simulink model "Rete"  (Simulink 9.0)
settings: Solver=VariableStepAuto  StartTime=0.0  StopTime=7200  RelTol=1e-3
values from neighbouring files (symbols this model uses):
  r_pompa = 100    [Circuit_configurator.m]
  vasca_1_r = 100    [Circuit_configurator.m]
  vasca_2_r = 100    [Circuit_configurator.m]
  vasca_3_r = 100    [Circuit_configurator.m]
  vasca_r_in = single(100)    [Circuit_configurator.m]
  vasca_sw = uint8(1)    [Circuit_configurator.m]
libraries: fl_lib x27, nesl_utility x24, elec_lib x8, realtime_pacer_lib x1
settings Model: SuppressorTable=22 serialization::archive 11 0 6 0 0 0 11 0  Creator=aleskandro  LastModifiedBy=aleskandro
settings DataIOCC: SaveFormat=Dataset
settings OptimizationCC: LifeSpan=auto
settings DebuggingCC: UnderspecifiedInitializationDetection=Simplified  MergeDetectMultiDrivingBlocksExec=error  SFUnexpectedBacktrackingDiag=error  SFNoUnconditionalDefaultTransitionDiag=error  SFExecutionAtInitializationDiag=warning
settings HardwareCC: ProdBitPerPointer=64  ProdBitPerSizeT=64  ProdBitPerPtrDiffT=64  ProdLargestAtomicFloat=Float  ProdIntDivRoundTo=Zero  ProdEndianess=LittleEndian  ProdWordSize=64  ProdHWDeviceType=Intel->x86-64 (Windows64)
settings ModelReferenceCC: PropagateSignalLabelsOutOfModel=on
settings GRTTargetCC: TargetLangStandard=C99 (ISO)
settings ConfigComp: CovMetricSettings=dwe  CovHtmlReporting=off  CovSaveCumulativeToWorkspaceVar=off  CovSaveSingleToWorkspaceVar=off  CovExternalEMLEnable=on
settings SimscapeCC: SimscapeNormalizeSystem=off

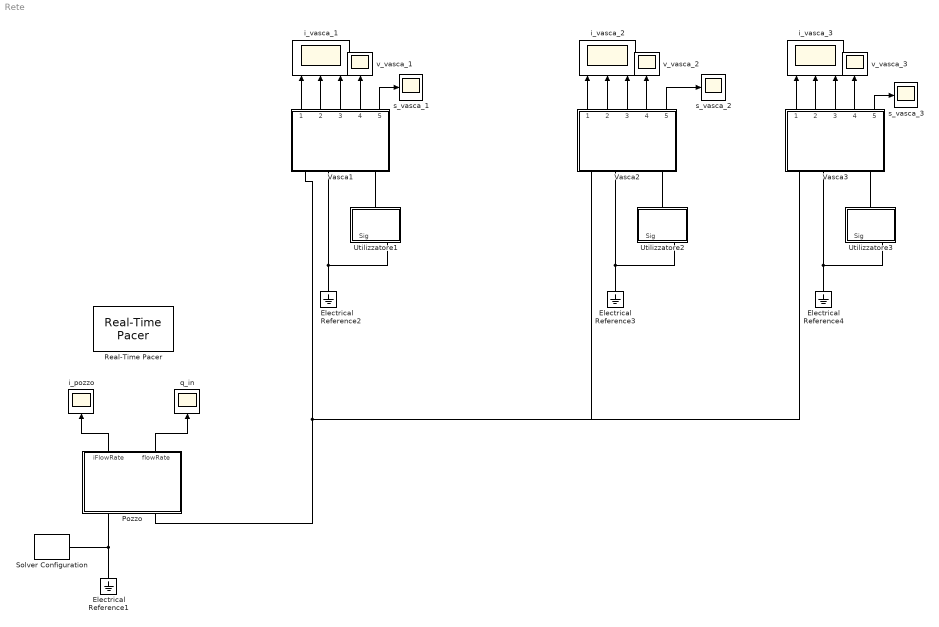
== system Rete ==
  Electrical Reference{1..4} (4 alike) : fl_lib/Electrical/Electrical Elements/Electrical Reference
  Pozzo : Subsystem
  Real-Time Pacer : realtime_pacer_lib/Real-Time Pacer  simTimePerRealTime=1
  Solver Configuration : nesl_utility/Solver Configuration  PhysicalDomain=network_engine_domain  SubClassName=solver  LeftPortType=input  RightPortType=generic  Accelerate=off  Tones=[]  Harmonics=[]  SimulateNoise=off  Profile=off  UseLocalSampling=off  EnableSwitchedLinearOptims=on  FrequencyDomain=off  UseCCode=off  RelTol=0.001  AbsTol=1e-06  MinStep=1e-09  ToWorkspace=off  RevertToSquareIcSolve=off  NumHomotopyIterations=100  PhasorMode=off  PhasorModeNumHarmonics=1  DoDC=off  ResidualTolerance=1e-09  UseLocalSolver=on  LocalSolverChoice=NE_BACKWARD_EULER_ADVANCER  LocalSolverSampleTime=0.1  DoFixedCost=on  MaxNonlinIter=3  MaxModeIter=2  LinearAlgebra=Sparse  DelaysMemoryBudget=1024  AutomaticFiltering=on  FilteringTimeConstant=0.001
  Utilizzatore1 : Subsystem
  Utilizzatore2 : Subsystem
  Utilizzatore3 : Subsystem
  Vasca1 : Subsystem
  Vasca2 : Subsystem
  Vasca3 : Subsystem
  i_pozzo : Scope
  i_vasca_1 : Scope  NumInputPorts=3
  i_vasca_2 : Scope  NumInputPorts=3
  i_vasca_3 : Scope  NumInputPorts=3
  q_in : Scope
  s_vasca_1 : Scope
  s_vasca_2 : Scope
  s_vasca_3 : Scope
  v_vasca_1 : Scope
  v_vasca_2 : Scope
  v_vasca_3 : Scope
  wires:
  Vasca1/4(vPression) -> v_vasca_1/1
  Pozzo/2(flowRate) -> q_in/1
  Pozzo/1(iFlowRate) -> i_pozzo/1
  Vasca1/2(flowRateOut) -> i_vasca_1/2
  Vasca1/1(flowRateIn) -> i_vasca_1/1
  Vasca1/3(vFlowRate) -> i_vasca_1/3
  Vasca2/3(vFlowRate) -> i_vasca_2/3
  Vasca2/4(vPression) -> v_vasca_2/1
  Vasca2/2(flowRateOut) -> i_vasca_2/2
  Vasca2/1(flowRateIn) -> i_vasca_2/1
  Vasca3/3(vFlowRate) -> i_vasca_3/3
  Vasca3/4(vPression) -> v_vasca_3/1
  Vasca3/2(flowRateOut) -> i_vasca_3/2
  Vasca3/1(flowRateIn) -> i_vasca_3/1
  Vasca2/5(switch) -> s_vasca_2/1
  Vasca3/5(switch) -> s_vasca_3/1
  Vasca1/5(switch) -> s_vasca_1/1
  connections:
  Electrical Reference1/LConn1 -- Solver Configuration/RConn1 -- Pozzo/LConn1
  Electrical Reference2/LConn1 -- Utilizzatore1/RConn1 -- Vasca1/LConn2
  Vasca1/LConn4 -- Utilizzatore1/LConn1
  Electrical Reference3/LConn1 -- Vasca2/LConn2 -- Utilizzatore2/RConn1
  Vasca2/LConn4 -- Utilizzatore2/LConn1
  Electrical Reference4/LConn1 -- Vasca3/LConn2 -- Utilizzatore3/RConn1
  Vasca3/LConn4 -- Utilizzatore3/LConn1
  Vasca3/LConn1 -- Vasca2/LConn1 -- Pozzo/LConn2 -- Vasca1/LConn1

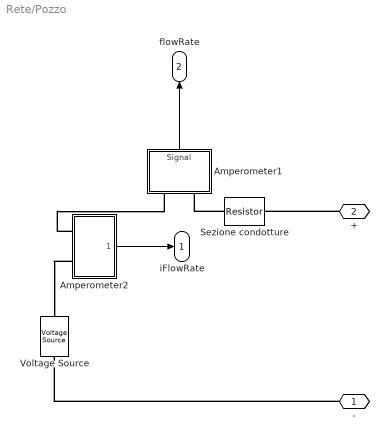
== system Rete/Pozzo ==
  Amperometer1 : Subsystem
  Amperometer2 : Subsystem
  Sezione condotture : elec_lib/Passive Devices/Resistor  R=r_pompa Ohm  R_tol=5  enable_R_tol=0  tol_distribution=1  nSigma=4  enable_operating_limits=0  operating_limit_action=2  max_working_voltage=100 V  power_rating=1 W  enable_faults=0  fault_action=1  R_faulted=Inf Ohm  enable_temporal_fault=0  t_fault=1 s  enable_behavioral_fault=0  max_permissible_current=1 A  t_fail_on_current=1 s  noise_mode=0  sample_time=0.001 s  repeatability=1  auto_seed=3797408467  user_seed=0  Tdevice=25 degC  alpha=3.93e-3 1/K  Tmeas=25 degC  thermal_mass=100 J/K  power_derating_T1=70 degC  power_derating_T2=155 degC  operating_temperature_range_vec=[-50, 150] degC  temperature_specify=off  temperature_priority=High  temperature=298.15 K  temperature_nominal_specify=off  temperature_nominal_unit=K  temperature_nominal_value=1
  Voltage Source : elec_lib/Sources/Voltage Source  dc_voltage=v_pompa V  ac_voltage=0 V  ac_shift=0 deg  ac_frequency=0 Hz  noise_mode=0  PSD=0 V^2/Hz  repeatability=1  auto_seed=2589191353  user_seed=0  sample_time=0.001 s  i_specify=off  i_priority=None  i=0 A  i_nominal_specify=off  i_nominal_unit=A  i_nominal_value=1  v_specify=off  v_priority=None  v=0 V  v_nominal_specify=off  v_nominal_unit=V  v_nominal_value=1
      settings: SourceProductName=Simscape Electronics  SourceProductBaseCode=SN
  - : PMIOPort  Port=1  Side=Left
  + : PMIOPort  Port=2  Side=Left
  iFlowRate : Outport
  flowRate : Outport  Port=2
  wires:
  Amperometer2/1(Signal) -> iFlowRate/1
  Amperometer1/1(Signal) -> flowRate/1
  connections:
  +/RConn1 -- Sezione condotture/RConn1
  -/RConn1 -- Voltage Source/RConn1
  Amperometer2/LConn2 -- Voltage Source/LConn1
  Amperometer2/LConn1 -- Amperometer1/LConn1
  Sezione condotture/LConn1 -- Amperometer1/LConn2

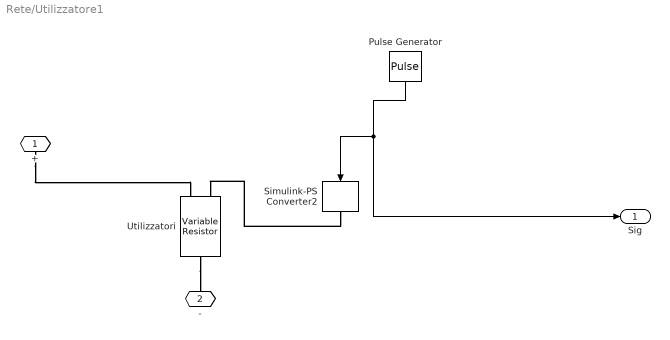
== system Rete/Utilizzatore1 ==
  Pulse Generator : DiscretePulseGenerator  Amplitude=999999999  Period=3000  PulseWidth=1500  PhaseDelay=4200
  Simulink-PS Converter2 : nesl_utility/Simulink-PS Converter  PhysicalDomain=network_engine_domain  SubClassName=ps_input  LeftPortType=input  RightPortType=output  PseudoPeriodic=off  Frequencies=[]  NoiseDistribution=none  NoiseParameters=[]  Unit=1  AffineConversion=off  FilteringAndDerivatives=zero  SimscapeFilterOrder=1  InputFilterTimeConstant=0.001  UdotUserProvided=1
  Utilizzatori : fl_lib/Electrical/Electrical Elements/Variable Resistor  Rmin=0 Ohm  i_specify=off  i_priority=High  i=0 A  i_nominal_specify=off  i_nominal_unit=A  i_nominal_value=1  v_specify=off  v_priority=High  v=0 V  v_nominal_specify=off  v_nominal_unit=V  v_nominal_value=1
  + : PMIOPort  Port=1  Side=Left
  - : PMIOPort  Port=2  Side=Right
  Sig : Outport
  wires:
  Pulse Generator/1 -> Sig/1, Simulink-PS Converter2/1
  connections:
  +/RConn1 -- Utilizzatori/LConn2
  Utilizzatori/RConn1 -- -/RConn1
  Simulink-PS Converter2/RConn1 -- Utilizzatori/LConn1

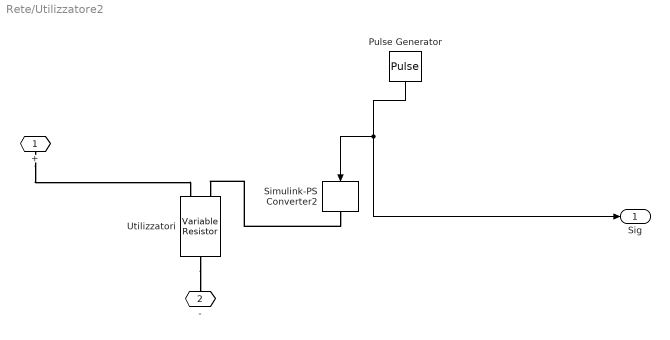
== system Rete/Utilizzatore2 ==
  Pulse Generator : DiscretePulseGenerator  Amplitude=999999999  Period=3000  PulseWidth=1500  PhaseDelay=4200
  Simulink-PS Converter2 : nesl_utility/Simulink-PS Converter  PhysicalDomain=network_engine_domain  SubClassName=ps_input  LeftPortType=input  RightPortType=output  PseudoPeriodic=off  Frequencies=[]  NoiseDistribution=none  NoiseParameters=[]  Unit=1  AffineConversion=off  FilteringAndDerivatives=zero  SimscapeFilterOrder=1  InputFilterTimeConstant=0.001  UdotUserProvided=1
  Utilizzatori : fl_lib/Electrical/Electrical Elements/Variable Resistor  Rmin=0 Ohm  i_specify=off  i_priority=High  i=0 A  i_nominal_specify=off  i_nominal_unit=A  i_nominal_value=1  v_specify=off  v_priority=High  v=0 V  v_nominal_specify=off  v_nominal_unit=V  v_nominal_value=1
  + : PMIOPort  Port=1  Side=Left
  - : PMIOPort  Port=2  Side=Right
  Sig : Outport
  wires:
  Pulse Generator/1 -> Sig/1, Simulink-PS Converter2/1
  connections:
  +/RConn1 -- Utilizzatori/LConn2
  Utilizzatori/RConn1 -- -/RConn1
  Simulink-PS Converter2/RConn1 -- Utilizzatori/LConn1

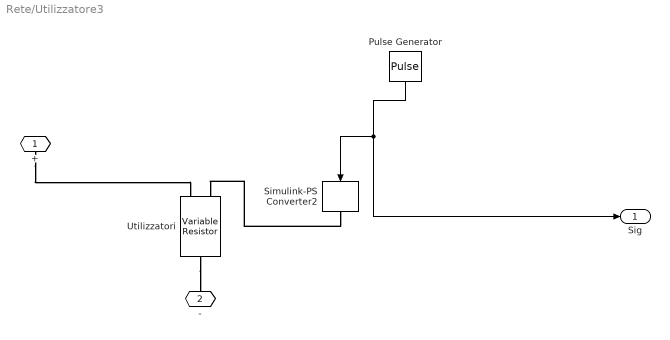
== system Rete/Utilizzatore3 ==
  Pulse Generator : DiscretePulseGenerator  Amplitude=999999999  Period=3000  PulseWidth=1500  PhaseDelay=4200
  Simulink-PS Converter2 : nesl_utility/Simulink-PS Converter  PhysicalDomain=network_engine_domain  SubClassName=ps_input  LeftPortType=input  RightPortType=output  PseudoPeriodic=off  Frequencies=[]  NoiseDistribution=none  NoiseParameters=[]  Unit=1  AffineConversion=off  FilteringAndDerivatives=zero  SimscapeFilterOrder=1  InputFilterTimeConstant=0.001  UdotUserProvided=1
  Utilizzatori : fl_lib/Electrical/Electrical Elements/Variable Resistor  Rmin=0 Ohm  i_specify=off  i_priority=High  i=0 A  i_nominal_specify=off  i_nominal_unit=A  i_nominal_value=1  v_specify=off  v_priority=High  v=0 V  v_nominal_specify=off  v_nominal_unit=V  v_nominal_value=1
  + : PMIOPort  Port=1  Side=Left
  - : PMIOPort  Port=2  Side=Right
  Sig : Outport
  wires:
  Pulse Generator/1 -> Sig/1, Simulink-PS Converter2/1
  connections:
  +/RConn1 -- Utilizzatori/LConn2
  Utilizzatori/RConn1 -- -/RConn1
  Simulink-PS Converter2/RConn1 -- Utilizzatori/LConn1

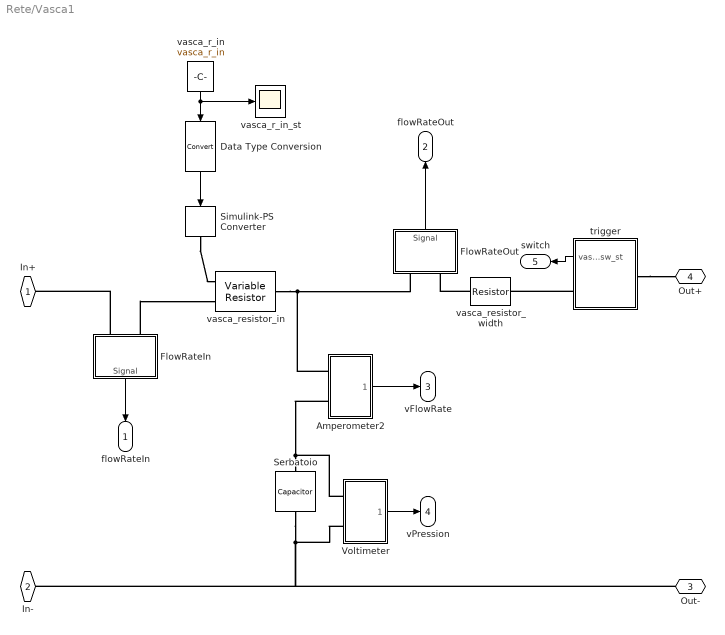
== system Rete/Vasca1 ==
  Amperometer2 : Subsystem
  Data Type Conversion : DataTypeConversion
  FlowRateIn : Subsystem
  FlowRateOut : Subsystem
  Serbatoio : elec_lib/Passive Devices/Capacitor  enable_table=0  c=vasca_1_c F  Cvec=[ 1e-5 1e-6 ] F  Vvec=[ 0 10 ] V  CV_table_symmetry=1  C_tol=5  enable_C_tol=0  tol_distribution=1  nSigma=4  r=1e-6 Ohm  g=0 1/Ohm  enable_operating_limits=0  operating_limit_action=2  max_working_voltage_range=[ -25 25 ] V  power_rating=1 W  enable_faults=0  fault_action=1  Cscale_faulted=100  R_faulted=0.001 Ohm  G_faulted=0 1/Ohm  tau_fault=0.001 s  enable_temporal_fault=0  t_fault=1 s  enable_behavioral_fault=0  max_permissible_voltage_range=[ -100 100 ] V  t_fail_on_voltage=1 s  i_specify=off  i_priority=None  i=0 A  i_nominal_specify=off  i_nominal_unit=A  i_nominal_value=1  v_specify=off  v_priority=None  v=0 V  v_nominal_specify=off  v_nominal_unit=V  v_nominal_value=1  vc_specify=on  vc_priority=High  vc=500 V  vc_nominal_specify=off  vc_nominal_unit=V  vc_nominal_value=1
  Simulink-PS Converter : nesl_utility/Simulink-PS Converter  PhysicalDomain=network_engine_domain  SubClassName=ps_input  LeftPortType=input  RightPortType=output  PseudoPeriodic=off  Frequencies=[]  NoiseDistribution=none  NoiseParameters=[]  Unit=1  AffineConversion=off  FilteringAndDerivatives=zero  SimscapeFilterOrder=1  InputFilterTimeConstant=0.001  UdotUserProvided=1
  Voltimeter : Subsystem
  trigger : Subsystem
  vasca_r_in : Constant  Value=vasca_r_in
  vasca_r_in_st : Scope
  vasca_resistor_in : fl_lib/Electrical/Electrical Elements/Variable Resistor  Rmin=0 Ohm  i_specify=off  i_priority=None  i=0 A  i_nominal_specify=off  i_nominal_unit=A  i_nominal_value=1  v_specify=off  v_priority=None  v=0 V  v_nominal_specify=off  v_nominal_unit=V  v_nominal_value=1
  vasca_resistor_width : elec_lib/Passive Devices/Resistor  R=vasca_1_r Ohm  R_tol=5  enable_R_tol=0  tol_distribution=1  nSigma=4  enable_operating_limits=0  operating_limit_action=2  max_working_voltage=100 V  power_rating=1 W  enable_faults=0  fault_action=1  R_faulted=Inf Ohm  enable_temporal_fault=0  t_fault=1 s  enable_behavioral_fault=0  max_permissible_current=1 A  t_fail_on_current=1 s  noise_mode=0  sample_time=0.001 s  repeatability=1  auto_seed=2536105935  user_seed=0  Tdevice=25 degC  alpha=3.93e-3 1/K  Tmeas=25 degC  thermal_mass=100 J/K  power_derating_T1=70 degC  power_derating_T2=155 degC  operating_temperature_range_vec=[-50, 150] degC  temperature_specify=off  temperature_priority=High  temperature=298.15 K  temperature_nominal_specify=off  temperature_nominal_unit=K  temperature_nominal_value=1
  In+ : PMIOPort  Port=1  Side=Left
  In- : PMIOPort  Port=2  Side=Left
  Out- : PMIOPort  Port=3  Side=Left
  Out+ : PMIOPort  Port=4  Side=Left
  flowRateIn : Outport
  flowRateOut : Outport  Port=2
  vFlowRate : Outport  Port=3
  vPression : Outport  Port=4
  switch : Outport  Port=5
  wires:
  Amperometer2/1(Signal) -> vFlowRate/1
  Voltimeter/1(Signal) -> vPression/1
  FlowRateOut/1(Signal) -> flowRateOut/1
  trigger/1(vasca_sw_st) -> switch/1
  Data Type Conversion/1 -> Simulink-PS Converter/1
  vasca_r_in/1 -> Data Type Conversion/1, vasca_r_in_st/1
  FlowRateIn/1(Signal) -> flowRateIn/1
  connections:
  Voltimeter/LConn2 -- Serbatoio/RConn1 -- Out-/RConn1 -- In-/RConn1
  Amperometer2/LConn2 -- Voltimeter/LConn1 -- Serbatoio/LConn1
  Amperometer2/LConn1 -- vasca_resistor_in/RConn1 -- FlowRateOut/LConn1
  vasca_resistor_width/LConn1 -- FlowRateOut/LConn2
  Simulink-PS Converter/RConn1 -- vasca_resistor_in/LConn1
  trigger/RConn1 -- vasca_resistor_width/RConn1
  trigger/LConn1 -- Out+/RConn1
  FlowRateIn/LConn1 -- In+/RConn1
  FlowRateIn/LConn2 -- vasca_resistor_in/LConn2

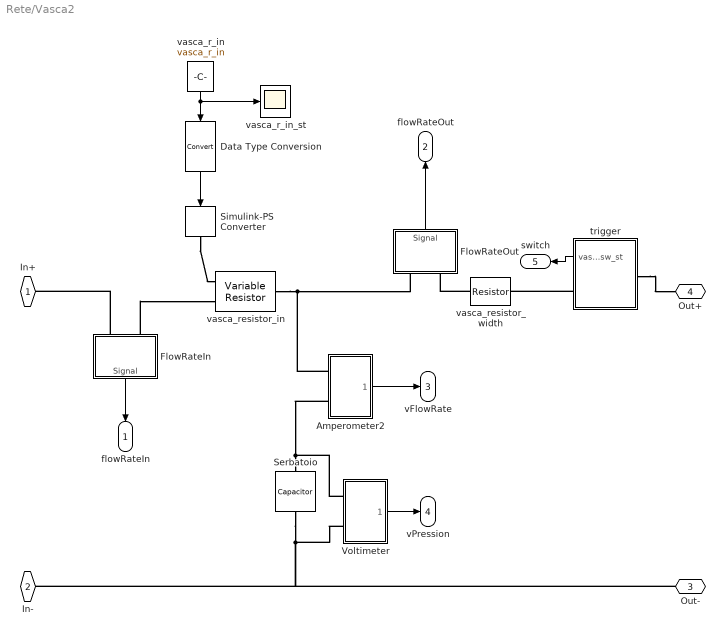
== system Rete/Vasca2 ==
  Amperometer2 : Subsystem
  Data Type Conversion : DataTypeConversion
  FlowRateIn : Subsystem
  FlowRateOut : Subsystem
  Serbatoio : elec_lib/Passive Devices/Capacitor  enable_table=0  c=vasca_2_c F  Cvec=[ 1e-5 1e-6 ] F  Vvec=[ 0 10 ] V  CV_table_symmetry=1  C_tol=5  enable_C_tol=0  tol_distribution=1  nSigma=4  r=1e-6 Ohm  g=0 1/Ohm  enable_operating_limits=0  operating_limit_action=2  max_working_voltage_range=[ -25 25 ] V  power_rating=1 W  enable_faults=0  fault_action=1  Cscale_faulted=100  R_faulted=0.001 Ohm  G_faulted=0 1/Ohm  tau_fault=0.001 s  enable_temporal_fault=0  t_fault=1 s  enable_behavioral_fault=0  max_permissible_voltage_range=[ -100 100 ] V  t_fail_on_voltage=1 s  i_specify=off  i_priority=None  i=0 A  i_nominal_specify=off  i_nominal_unit=A  i_nominal_value=1  v_specify=off  v_priority=None  v=0 V  v_nominal_specify=off  v_nominal_unit=V  v_nominal_value=1  vc_specify=on  vc_priority=High  vc=500 V  vc_nominal_specify=off  vc_nominal_unit=V  vc_nominal_value=1
  Simulink-PS Converter : nesl_utility/Simulink-PS Converter  PhysicalDomain=network_engine_domain  SubClassName=ps_input  LeftPortType=input  RightPortType=output  PseudoPeriodic=off  Frequencies=[]  NoiseDistribution=none  NoiseParameters=[]  Unit=1  AffineConversion=off  FilteringAndDerivatives=zero  SimscapeFilterOrder=1  InputFilterTimeConstant=0.001  UdotUserProvided=1
  Voltimeter : Subsystem
  trigger : Subsystem
  vasca_r_in : Constant  Value=vasca_r_in
  vasca_r_in_st : Scope
  vasca_resistor_in : fl_lib/Electrical/Electrical Elements/Variable Resistor  Rmin=0 Ohm  i_specify=off  i_priority=None  i=0 A  i_nominal_specify=off  i_nominal_unit=A  i_nominal_value=1  v_specify=off  v_priority=None  v=0 V  v_nominal_specify=off  v_nominal_unit=V  v_nominal_value=1
  vasca_resistor_width : elec_lib/Passive Devices/Resistor  R=vasca_2_r Ohm  R_tol=5  enable_R_tol=0  tol_distribution=1  nSigma=4  enable_operating_limits=0  operating_limit_action=2  max_working_voltage=100 V  power_rating=1 W  enable_faults=0  fault_action=1  R_faulted=Inf Ohm  enable_temporal_fault=0  t_fault=1 s  enable_behavioral_fault=0  max_permissible_current=1 A  t_fail_on_current=1 s  noise_mode=0  sample_time=0.001 s  repeatability=1  auto_seed=2664075559  user_seed=0  Tdevice=25 degC  alpha=3.93e-3 1/K  Tmeas=25 degC  thermal_mass=100 J/K  power_derating_T1=70 degC  power_derating_T2=155 degC  operating_temperature_range_vec=[-50, 150] degC  temperature_specify=off  temperature_priority=High  temperature=298.15 K  temperature_nominal_specify=off  temperature_nominal_unit=K  temperature_nominal_value=1
  In+ : PMIOPort  Port=1  Side=Left
  In- : PMIOPort  Port=2  Side=Left
  Out- : PMIOPort  Port=3  Side=Left
  Out+ : PMIOPort  Port=4  Side=Left
  flowRateIn : Outport
  flowRateOut : Outport  Port=2
  vFlowRate : Outport  Port=3
  vPression : Outport  Port=4
  switch : Outport  Port=5
  wires:
  Amperometer2/1(Signal) -> vFlowRate/1
  Voltimeter/1(Signal) -> vPression/1
  FlowRateOut/1(Signal) -> flowRateOut/1
  trigger/1(vasca_sw_st) -> switch/1
  Data Type Conversion/1 -> Simulink-PS Converter/1
  FlowRateIn/1(Signal) -> flowRateIn/1
  vasca_r_in/1 -> vasca_r_in_st/1, Data Type Conversion/1
  connections:
  Voltimeter/LConn2 -- Serbatoio/RConn1 -- Out-/RConn1 -- In-/RConn1
  Amperometer2/LConn2 -- Voltimeter/LConn1 -- Serbatoio/LConn1
  Amperometer2/LConn1 -- vasca_resistor_in/RConn1 -- FlowRateOut/LConn1
  vasca_resistor_width/LConn1 -- FlowRateOut/LConn2
  Simulink-PS Converter/RConn1 -- vasca_resistor_in/LConn1
  trigger/RConn1 -- vasca_resistor_width/RConn1
  trigger/LConn1 -- Out+/RConn1
  FlowRateIn/LConn1 -- In+/RConn1
  FlowRateIn/LConn2 -- vasca_resistor_in/LConn2

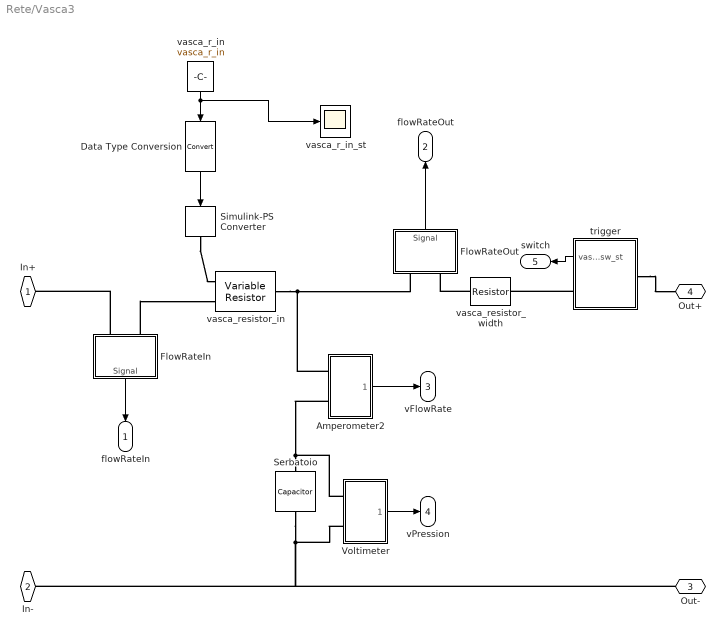
== system Rete/Vasca3 ==
  Amperometer2 : Subsystem
  Data Type Conversion : DataTypeConversion
  FlowRateIn : Subsystem
  FlowRateOut : Subsystem
  Serbatoio : elec_lib/Passive Devices/Capacitor  enable_table=0  c=vasca_3_c F  Cvec=[ 1e-5 1e-6 ] F  Vvec=[ 0 10 ] V  CV_table_symmetry=1  C_tol=5  enable_C_tol=0  tol_distribution=1  nSigma=4  r=1e-6 Ohm  g=0 1/Ohm  enable_operating_limits=0  operating_limit_action=2  max_working_voltage_range=[ -25 25 ] V  power_rating=1 W  enable_faults=0  fault_action=1  Cscale_faulted=100  R_faulted=0.001 Ohm  G_faulted=0 1/Ohm  tau_fault=0.001 s  enable_temporal_fault=0  t_fault=1 s  enable_behavioral_fault=0  max_permissible_voltage_range=[ -100 100 ] V  t_fail_on_voltage=1 s  i_specify=off  i_priority=None  i=0 A  i_nominal_specify=off  i_nominal_unit=A  i_nominal_value=1  v_specify=off  v_priority=None  v=0 V  v_nominal_specify=off  v_nominal_unit=V  v_nominal_value=1  vc_specify=on  vc_priority=High  vc=500 V  vc_nominal_specify=off  vc_nominal_unit=V  vc_nominal_value=1
  Simulink-PS Converter : nesl_utility/Simulink-PS Converter  PhysicalDomain=network_engine_domain  SubClassName=ps_input  LeftPortType=input  RightPortType=output  PseudoPeriodic=off  Frequencies=[]  NoiseDistribution=none  NoiseParameters=[]  Unit=1  AffineConversion=off  FilteringAndDerivatives=zero  SimscapeFilterOrder=1  InputFilterTimeConstant=0.001  UdotUserProvided=1
  Voltimeter : Subsystem
  trigger : Subsystem
  vasca_r_in : Constant  Value=vasca_r_in
  vasca_r_in_st : Scope
  vasca_resistor_in : fl_lib/Electrical/Electrical Elements/Variable Resistor  Rmin=0 Ohm  i_specify=off  i_priority=None  i=0 A  i_nominal_specify=off  i_nominal_unit=A  i_nominal_value=1  v_specify=off  v_priority=None  v=0 V  v_nominal_specify=off  v_nominal_unit=V  v_nominal_value=1
  vasca_resistor_width : elec_lib/Passive Devices/Resistor  R=vasca_3_r Ohm  R_tol=5  enable_R_tol=0  tol_distribution=1  nSigma=4  enable_operating_limits=0  operating_limit_action=2  max_working_voltage=100 V  power_rating=1 W  enable_faults=0  fault_action=1  R_faulted=Inf Ohm  enable_temporal_fault=0  t_fault=1 s  enable_behavioral_fault=0  max_permissible_current=1 A  t_fail_on_current=1 s  noise_mode=0  sample_time=0.001 s  repeatability=1  auto_seed=82710236  user_seed=0  Tdevice=25 degC  alpha=3.93e-3 1/K  Tmeas=25 degC  thermal_mass=100 J/K  power_derating_T1=70 degC  power_derating_T2=155 degC  operating_temperature_range_vec=[-50, 150] degC  temperature_specify=off  temperature_priority=High  temperature=298.15 K  temperature_nominal_specify=off  temperature_nominal_unit=K  temperature_nominal_value=1
  In+ : PMIOPort  Port=1  Side=Left
  In- : PMIOPort  Port=2  Side=Left
  Out- : PMIOPort  Port=3  Side=Left
  Out+ : PMIOPort  Port=4  Side=Left
  flowRateIn : Outport
  flowRateOut : Outport  Port=2
  vFlowRate : Outport  Port=3
  vPression : Outport  Port=4
  switch : Outport  Port=5
  wires:
  Amperometer2/1(Signal) -> vFlowRate/1
  Voltimeter/1(Signal) -> vPression/1
  FlowRateOut/1(Signal) -> flowRateOut/1
  trigger/1(vasca_sw_st) -> switch/1
  Data Type Conversion/1 -> Simulink-PS Converter/1
  FlowRateIn/1(Signal) -> flowRateIn/1
  vasca_r_in/1 -> vasca_r_in_st/1, Data Type Conversion/1
  connections:
  Voltimeter/LConn2 -- Serbatoio/RConn1 -- Out-/RConn1 -- In-/RConn1
  Amperometer2/LConn2 -- Voltimeter/LConn1 -- Serbatoio/LConn1
  Amperometer2/LConn1 -- vasca_resistor_in/RConn1 -- FlowRateOut/LConn1
  vasca_resistor_width/LConn1 -- FlowRateOut/LConn2
  Simulink-PS Converter/RConn1 -- vasca_resistor_in/LConn1
  trigger/RConn1 -- vasca_resistor_width/RConn1
  trigger/LConn1 -- Out+/RConn1
  FlowRateIn/LConn1 -- In+/RConn1
  FlowRateIn/LConn2 -- vasca_resistor_in/LConn2

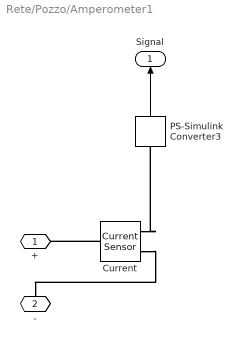
== system Rete/Pozzo/Amperometer1 ==
  Current : fl_lib/Electrical/Electrical Sensors/Current Sensor
  PS-Simulink Converter3 : nesl_utility/PS-Simulink Converter  PhysicalDomain=network_engine_domain  SubClassName=ps_output  LeftPortType=input  RightPortType=output  PseudoPeriodic=off  Frequencies=[]  Unit=A  AffineConversion=off
  "+ " : PMIOPort  Port=1  Side=Left
  - : PMIOPort  Port=2  Side=Left
  Signal : Outport
  wires:
  PS-Simulink Converter3/1 -> Signal/1
  connections:
  Current/RConn1 -- PS-Simulink Converter3/LConn1
  Current/RConn2 -- -/RConn1
  Current/LConn1 -- "+ "/RConn1

== system Rete/Pozzo/Amperometer2 ==
  Current : fl_lib/Electrical/Electrical Sensors/Current Sensor
  PS-Simulink Converter3 : nesl_utility/PS-Simulink Converter  PhysicalDomain=network_engine_domain  SubClassName=ps_output  LeftPortType=input  RightPortType=output  PseudoPeriodic=off  Frequencies=[]  Unit=A  AffineConversion=off
  "+ " : PMIOPort  Port=1  Side=Left
  - : PMIOPort  Port=2  Side=Left
  Signal : Outport
  wires:
  PS-Simulink Converter3/1 -> Signal/1
  connections:
  Current/RConn1 -- PS-Simulink Converter3/LConn1
  Current/RConn2 -- -/RConn1
  Current/LConn1 -- "+ "/RConn1

== system Rete/Vasca1/Amperometer2 ==
  Current : fl_lib/Electrical/Electrical Sensors/Current Sensor
  PS-Simulink Converter3 : nesl_utility/PS-Simulink Converter  PhysicalDomain=network_engine_domain  SubClassName=ps_output  LeftPortType=input  RightPortType=output  PseudoPeriodic=off  Frequencies=[]  Unit=A  AffineConversion=off
  "+ " : PMIOPort  Port=1  Side=Left
  - : PMIOPort  Port=2  Side=Left
  Signal : Outport
  wires:
  PS-Simulink Converter3/1 -> Signal/1
  connections:
  Current/RConn1 -- PS-Simulink Converter3/LConn1
  Current/RConn2 -- -/RConn1
  Current/LConn1 -- "+ "/RConn1

== system Rete/Vasca1/FlowRateIn ==
  Current : fl_lib/Electrical/Electrical Sensors/Current Sensor
  PS-Simulink Converter3 : nesl_utility/PS-Simulink Converter  PhysicalDomain=network_engine_domain  SubClassName=ps_output  LeftPortType=input  RightPortType=output  PseudoPeriodic=off  Frequencies=[]  Unit=A  AffineConversion=off
  "+ " : PMIOPort  Port=1  Side=Left
  - : PMIOPort  Port=2  Side=Left
  Signal : Outport
  wires:
  PS-Simulink Converter3/1 -> Signal/1
  connections:
  Current/RConn1 -- PS-Simulink Converter3/LConn1
  Current/RConn2 -- -/RConn1
  Current/LConn1 -- "+ "/RConn1

== system Rete/Vasca1/FlowRateOut ==
  Current : fl_lib/Electrical/Electrical Sensors/Current Sensor
  Current1 : nesl_utility/PS-Simulink Converter  PhysicalDomain=network_engine_domain  SubClassName=ps_output  LeftPortType=input  RightPortType=output  PseudoPeriodic=off  Frequencies=[]  Unit=A  AffineConversion=off
  "+ " : PMIOPort  Port=1  Side=Left
  - : PMIOPort  Port=2  Side=Left
  Signal : Outport
  wires:
  Current1/1 -> Signal/1
  connections:
  Current/RConn1 -- Current1/LConn1
  Current/RConn2 -- -/RConn1
  Current/LConn1 -- "+ "/RConn1

== system Rete/Vasca1/Voltimeter ==
  PS-Simulink Converter4 : nesl_utility/PS-Simulink Converter  PhysicalDomain=network_engine_domain  SubClassName=ps_output  LeftPortType=input  RightPortType=output  PseudoPeriodic=off  Frequencies=[]  Unit=V  AffineConversion=off
  v_vasca1 : fl_lib/Electrical/Electrical Sensors/Voltage Sensor
  + : PMIOPort  Port=1  Side=Left
  - : PMIOPort  Port=2  Side=Left
  Signal : Outport
  wires:
  PS-Simulink Converter4/1 -> Signal/1
  connections:
  v_vasca1/LConn1 -- +/RConn1
  v_vasca1/RConn2 -- -/RConn1
  v_vasca1/RConn1 -- PS-Simulink Converter4/LConn1

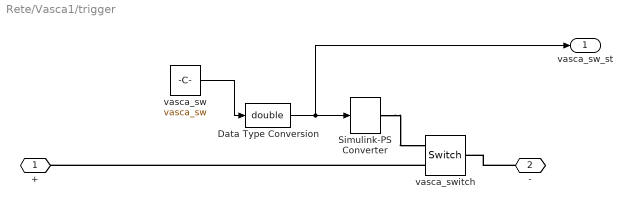
== system Rete/Vasca1/trigger ==
  Data Type Conversion : DataTypeConversion  OutDataTypeStr=double
  Simulink-PS Converter : nesl_utility/Simulink-PS Converter  PhysicalDomain=network_engine_domain  SubClassName=ps_input  LeftPortType=input  RightPortType=output  PseudoPeriodic=off  Frequencies=[]  NoiseDistribution=none  NoiseParameters=[]  Unit=1  AffineConversion=off  FilteringAndDerivatives=zero  SimscapeFilterOrder=1  InputFilterTimeConstant=0.001  UdotUserProvided=1
  vasca_sw : Constant  Value=vasca_sw  OutDataTypeStr=uint8
  vasca_switch : fl_lib/Electrical/Electrical Elements/Switch  R_closed=0.01 Ohm  G_open=1e-8 1/Ohm  Threshold=0.5  i_specify=off  i_priority=High  i=0 A  i_nominal_specify=off  i_nominal_unit=A  i_nominal_value=1  v_specify=off  v_priority=High  v=0 V  v_nominal_specify=off  v_nominal_unit=V  v_nominal_value=1
      settings: SourceProductName=Simscape
  + : PMIOPort  Port=1  Side=Right
  - : PMIOPort  Port=2  Side=Left
  vasca_sw_st : Outport
  wires:
  Data Type Conversion/1 -> vasca_sw_st/1, Simulink-PS Converter/1
  vasca_sw/1 -> Data Type Conversion/1
  connections:
  vasca_switch/RConn2 -- +/RConn1
  -/RConn1 -- vasca_switch/LConn1
  Simulink-PS Converter/RConn1 -- vasca_switch/RConn1

== system Rete/Vasca2/Amperometer2 ==
  Current : fl_lib/Electrical/Electrical Sensors/Current Sensor
  PS-Simulink Converter3 : nesl_utility/PS-Simulink Converter  PhysicalDomain=network_engine_domain  SubClassName=ps_output  LeftPortType=input  RightPortType=output  PseudoPeriodic=off  Frequencies=[]  Unit=A  AffineConversion=off
  "+ " : PMIOPort  Port=1  Side=Left
  - : PMIOPort  Port=2  Side=Left
  Signal : Outport
  wires:
  PS-Simulink Converter3/1 -> Signal/1
  connections:
  Current/RConn1 -- PS-Simulink Converter3/LConn1
  Current/RConn2 -- -/RConn1
  Current/LConn1 -- "+ "/RConn1

== system Rete/Vasca2/FlowRateIn ==
  Current : fl_lib/Electrical/Electrical Sensors/Current Sensor
  PS-Simulink Converter3 : nesl_utility/PS-Simulink Converter  PhysicalDomain=network_engine_domain  SubClassName=ps_output  LeftPortType=input  RightPortType=output  PseudoPeriodic=off  Frequencies=[]  Unit=A  AffineConversion=off
  "+ " : PMIOPort  Port=1  Side=Left
  - : PMIOPort  Port=2  Side=Left
  Signal : Outport
  wires:
  PS-Simulink Converter3/1 -> Signal/1
  connections:
  Current/RConn1 -- PS-Simulink Converter3/LConn1
  Current/RConn2 -- -/RConn1
  Current/LConn1 -- "+ "/RConn1

== system Rete/Vasca2/FlowRateOut ==
  Current : fl_lib/Electrical/Electrical Sensors/Current Sensor
  Current1 : nesl_utility/PS-Simulink Converter  PhysicalDomain=network_engine_domain  SubClassName=ps_output  LeftPortType=input  RightPortType=output  PseudoPeriodic=off  Frequencies=[]  Unit=A  AffineConversion=off
  "+ " : PMIOPort  Port=1  Side=Left
  - : PMIOPort  Port=2  Side=Left
  Signal : Outport
  wires:
  Current1/1 -> Signal/1
  connections:
  Current/RConn1 -- Current1/LConn1
  Current/RConn2 -- -/RConn1
  Current/LConn1 -- "+ "/RConn1

== system Rete/Vasca2/Voltimeter ==
  PS-Simulink Converter4 : nesl_utility/PS-Simulink Converter  PhysicalDomain=network_engine_domain  SubClassName=ps_output  LeftPortType=input  RightPortType=output  PseudoPeriodic=off  Frequencies=[]  Unit=V  AffineConversion=off
  v_vasca1 : fl_lib/Electrical/Electrical Sensors/Voltage Sensor
  + : PMIOPort  Port=1  Side=Left
  - : PMIOPort  Port=2  Side=Left
  Signal : Outport
  wires:
  PS-Simulink Converter4/1 -> Signal/1
  connections:
  v_vasca1/LConn1 -- +/RConn1
  v_vasca1/RConn2 -- -/RConn1
  v_vasca1/RConn1 -- PS-Simulink Converter4/LConn1

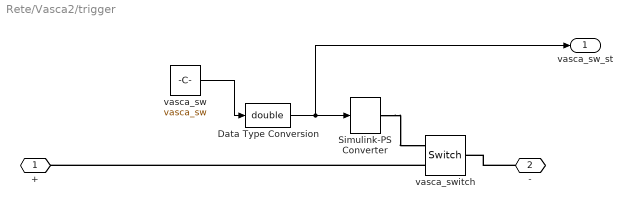
== system Rete/Vasca2/trigger ==
  Data Type Conversion : DataTypeConversion  OutDataTypeStr=double
  Simulink-PS Converter : nesl_utility/Simulink-PS Converter  PhysicalDomain=network_engine_domain  SubClassName=ps_input  LeftPortType=input  RightPortType=output  PseudoPeriodic=off  Frequencies=[]  NoiseDistribution=none  NoiseParameters=[]  Unit=1  AffineConversion=off  FilteringAndDerivatives=zero  SimscapeFilterOrder=1  InputFilterTimeConstant=0.001  UdotUserProvided=1
  vasca_sw : Constant  Value=vasca_sw  OutDataTypeStr=uint8
  vasca_switch : fl_lib/Electrical/Electrical Elements/Switch  R_closed=0.01 Ohm  G_open=1e-8 1/Ohm  Threshold=0.5  i_specify=off  i_priority=High  i=0 A  i_nominal_specify=off  i_nominal_unit=A  i_nominal_value=1  v_specify=off  v_priority=High  v=0 V  v_nominal_specify=off  v_nominal_unit=V  v_nominal_value=1
      settings: SourceProductName=Simscape
  + : PMIOPort  Port=1  Side=Right
  - : PMIOPort  Port=2  Side=Left
  vasca_sw_st : Outport
  wires:
  Data Type Conversion/1 -> vasca_sw_st/1, Simulink-PS Converter/1
  vasca_sw/1 -> Data Type Conversion/1
  connections:
  vasca_switch/RConn2 -- +/RConn1
  -/RConn1 -- vasca_switch/LConn1
  Simulink-PS Converter/RConn1 -- vasca_switch/RConn1

== system Rete/Vasca3/Amperometer2 ==
  Current : fl_lib/Electrical/Electrical Sensors/Current Sensor
  PS-Simulink Converter3 : nesl_utility/PS-Simulink Converter  PhysicalDomain=network_engine_domain  SubClassName=ps_output  LeftPortType=input  RightPortType=output  PseudoPeriodic=off  Frequencies=[]  Unit=A  AffineConversion=off
  "+ " : PMIOPort  Port=1  Side=Left
  - : PMIOPort  Port=2  Side=Left
  Signal : Outport
  wires:
  PS-Simulink Converter3/1 -> Signal/1
  connections:
  Current/RConn1 -- PS-Simulink Converter3/LConn1
  Current/RConn2 -- -/RConn1
  Current/LConn1 -- "+ "/RConn1

== system Rete/Vasca3/FlowRateIn ==
  Current : fl_lib/Electrical/Electrical Sensors/Current Sensor
  PS-Simulink Converter3 : nesl_utility/PS-Simulink Converter  PhysicalDomain=network_engine_domain  SubClassName=ps_output  LeftPortType=input  RightPortType=output  PseudoPeriodic=off  Frequencies=[]  Unit=A  AffineConversion=off
  "+ " : PMIOPort  Port=1  Side=Left
  - : PMIOPort  Port=2  Side=Left
  Signal : Outport
  wires:
  PS-Simulink Converter3/1 -> Signal/1
  connections:
  Current/RConn1 -- PS-Simulink Converter3/LConn1
  Current/RConn2 -- -/RConn1
  Current/LConn1 -- "+ "/RConn1

== system Rete/Vasca3/FlowRateOut ==
  Current : fl_lib/Electrical/Electrical Sensors/Current Sensor
  Current1 : nesl_utility/PS-Simulink Converter  PhysicalDomain=network_engine_domain  SubClassName=ps_output  LeftPortType=input  RightPortType=output  PseudoPeriodic=off  Frequencies=[]  Unit=A  AffineConversion=off
  "+ " : PMIOPort  Port=1  Side=Left
  - : PMIOPort  Port=2  Side=Left
  Signal : Outport
  wires:
  Current1/1 -> Signal/1
  connections:
  Current/RConn1 -- Current1/LConn1
  Current/RConn2 -- -/RConn1
  Current/LConn1 -- "+ "/RConn1

== system Rete/Vasca3/Voltimeter ==
  PS-Simulink Converter4 : nesl_utility/PS-Simulink Converter  PhysicalDomain=network_engine_domain  SubClassName=ps_output  LeftPortType=input  RightPortType=output  PseudoPeriodic=off  Frequencies=[]  Unit=V  AffineConversion=off
  v_vasca1 : fl_lib/Electrical/Electrical Sensors/Voltage Sensor
  + : PMIOPort  Port=1  Side=Left
  - : PMIOPort  Port=2  Side=Left
  Signal : Outport
  wires:
  PS-Simulink Converter4/1 -> Signal/1
  connections:
  v_vasca1/LConn1 -- +/RConn1
  v_vasca1/RConn2 -- -/RConn1
  v_vasca1/RConn1 -- PS-Simulink Converter4/LConn1

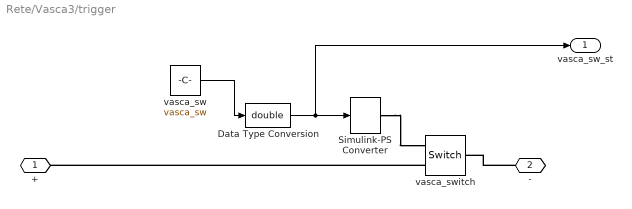
== system Rete/Vasca3/trigger ==
  Data Type Conversion : DataTypeConversion  OutDataTypeStr=double
  Simulink-PS Converter : nesl_utility/Simulink-PS Converter  PhysicalDomain=network_engine_domain  SubClassName=ps_input  LeftPortType=input  RightPortType=output  PseudoPeriodic=off  Frequencies=[]  NoiseDistribution=none  NoiseParameters=[]  Unit=1  AffineConversion=off  FilteringAndDerivatives=zero  SimscapeFilterOrder=1  InputFilterTimeConstant=0.001  UdotUserProvided=1
  vasca_sw : Constant  Value=vasca_sw  OutDataTypeStr=uint8
  vasca_switch : fl_lib/Electrical/Electrical Elements/Switch  R_closed=0.01 Ohm  G_open=1e-8 1/Ohm  Threshold=0.5  i_specify=off  i_priority=High  i=0 A  i_nominal_specify=off  i_nominal_unit=A  i_nominal_value=1  v_specify=off  v_priority=High  v=0 V  v_nominal_specify=off  v_nominal_unit=V  v_nominal_value=1
      settings: SourceProductName=Simscape
  + : PMIOPort  Port=1  Side=Right
  - : PMIOPort  Port=2  Side=Left
  vasca_sw_st : Outport
  wires:
  Data Type Conversion/1 -> vasca_sw_st/1, Simulink-PS Converter/1
  vasca_sw/1 -> Data Type Conversion/1
  connections:
  vasca_switch/RConn2 -- +/RConn1
  -/RConn1 -- vasca_switch/LConn1
  Simulink-PS Converter/RConn1 -- vasca_switch/RConn1
